simulink model "TCC_MODEL"  (R2025a)
settings: Solver=ode23t  StartTime=0.0  StopTime=1010  FixedStep=0.01  RelTol=1e-3
values from neighbouring files (symbols this model uses):
  HYST = 2    [parametros_componentes.m]
  I_table = [  1.6305773075253425 ... (first row only)    [parametros_componentes.m]
  Icc = -0.000008    (= -8e-06)    [parametros_componentes.m]
  IDD = 25e-6    (= 2.5e-05)    [parametros_componentes.m]
  Ildo = -0.00007    (= -7e-05)    [parametros_componentes.m]
  Iload = 0    [parametros_componentes.m]
  Inicio_da_descarga = 1000    [parametros_componentes.m]
  Inicio_do_curto = 10    [parametros_componentes.m]
  R_curto = 0.5    [parametros_componentes.m]
  R_descarga = (V_BATT_TOTAL+12)/corrente_Max_bat    (= 8.05)    [parametros_componentes.m]
  R_inicial = 0.18    [parametros_componentes.m]
  R_trip = 64.8    [parametros_componentes.m]
  SOC_inicial = 1    [parametros_componentes.m]
  t_table = [  93.22913720326267 ... (first row only)    [parametros_componentes.m]
  tempo_simu_curto = 70    [parametros_componentes.m]
  tempo_simu_descarga = 20    [parametros_componentes.m]
  tempo_simu_temp = 50000    [parametros_componentes.m]
  TSET = 55    [parametros_componentes.m]
  VDD = 3.3    [parametros_componentes.m]
libraries: fl_lib x29, nesl_utility x21, batt_lib x12, ee_lib x2, simulink x1, BatteryEstimators x1
(part 2 of 2)

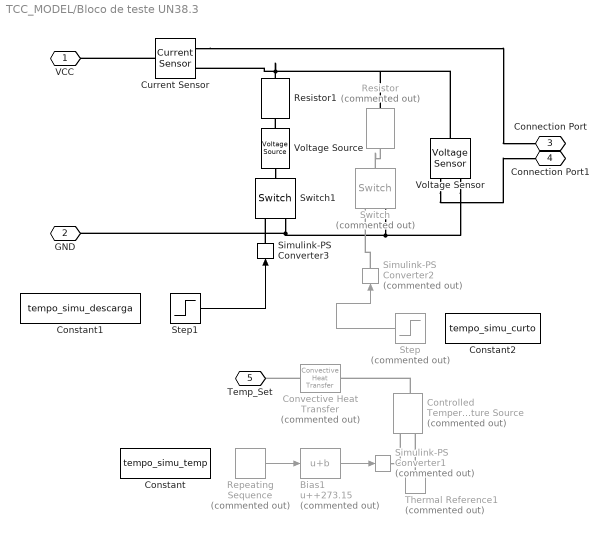
== system TCC_MODEL/Bloco de teste UN38.3 ==
  Bias1 : Bias  Commented=on  Bias=+273.15  SaturateOnIntegerOverflow=off
  Constant : Constant  Value=tempo_simu_temp
  Constant1 : Constant  Value=tempo_simu_descarga
  Constant2 : Constant  Value=tempo_simu_curto
  Controlled Temperature Source : fl_lib/Thermal/Thermal Sources/Controlled Temperature Source  Commented=on
  Convective Heat Transfer : fl_lib/Thermal/Thermal Elements/Convective Heat Transfer  Commented=on  thermal_type=foundation.enum.constant_variable.constant  area=0.03 m^2  heat_tr_coeff=10 W/(K*m^2)  min_heat_tr_coeff=1e-3 W/(K*m^2)  T_specify=off  T_priority=None  T=0 K  T_nominal_specify=off  T_nominal_value=1  T_nominal_unit=K  Q_specify=off  Q_priority=None  Q=0 W  Q_nominal_specify=off  Q_nominal_value=1  Q_nominal_unit=W
  Current Sensor : fl_lib/Electrical/Electrical Sensors/Current Sensor
  Repeating Sequence : simulink/Sources/Repeating Sequence  Commented=on  rep_seq_t=Tempo_de_teste  rep_seq_y=Valores_Temperatura
  Resistor : fl_lib/Electrical/Electrical Elements/Resistor  Commented=on  R=R_curto Ohm  i_specify=off  i_priority=None  i=0 A  i_nominal_specify=off  i_nominal_value=1  i_nominal_unit=A  v_specify=off  v_priority=None  v=0 V  v_nominal_specify=off  v_nominal_value=1  v_nominal_unit=V
  Resistor1 : fl_lib/Electrical/Electrical Elements/Resistor  R=R_descarga Ohm  i_specify=off  i_priority=None  i=0 A  i_nominal_specify=off  i_nominal_value=1  i_nominal_unit=A  v_specify=off  v_priority=None  v=0 V  v_nominal_specify=off  v_nominal_value=1  v_nominal_unit=V
  Simulink-PS Converter1 : nesl_utility/Simulink-PS Converter  Commented=on  PhysicalDomain=network_engine_domain  SubClassName=ps_input  LeftPortType=input  RightPortType=output  PseudoPeriodic=off  Frequencies=[]  NoiseDistribution=none  NoiseParameters=[]  Unit=1  AffineConversion=off  FilteringAndDerivatives=provide  SimscapeFilterOrder=1  InputFilterTimeConstant=0.001  UdotUserProvided=0
  Simulink-PS Converter2 : nesl_utility/Simulink-PS Converter  Commented=on  PhysicalDomain=network_engine_domain  SubClassName=ps_input  LeftPortType=input  RightPortType=output  PseudoPeriodic=off  Frequencies=[]  NoiseDistribution=none  NoiseParameters=[]  Unit=1  AffineConversion=off  FilteringAndDerivatives=provide  SimscapeFilterOrder=1  InputFilterTimeConstant=0.001  UdotUserProvided=0
  Simulink-PS Converter3 : nesl_utility/Simulink-PS Converter  PhysicalDomain=network_engine_domain  SubClassName=ps_input  LeftPortType=input  RightPortType=output  PseudoPeriodic=off  Frequencies=[]  NoiseDistribution=none  NoiseParameters=[]  Unit=1  AffineConversion=off  FilteringAndDerivatives=provide  SimscapeFilterOrder=1  InputFilterTimeConstant=0.001  UdotUserProvided=0
  Step : Step  Commented=on  Time=Inicio_do_curto  SampleTime=0
  Step1 : Step  Time=Inicio_da_descarga  SampleTime=0
  Switch : fl_lib/Electrical/Electrical Elements/Switch  Commented=on  R_closed=0.01 Ohm  G_open=1e-8 1/Ohm  Threshold=0.5  i_specify=off  i_priority=None  i=0 A  i_nominal_specify=off  i_nominal_value=1  i_nominal_unit=A  v_specify=off  v_priority=None  v=0 V  v_nominal_specify=off  v_nominal_value=1  v_nominal_unit=V
  Switch1 : fl_lib/Electrical/Electrical Elements/Switch  R_closed=0.01 Ohm  G_open=1e-8 1/Ohm  Threshold=0.5  i_specify=off  i_priority=None  i=0 A  i_nominal_specify=off  i_nominal_value=1  i_nominal_unit=A  v_specify=off  v_priority=None  v=0 V  v_nominal_specify=off  v_nominal_value=1  v_nominal_unit=V
  Thermal Reference1 : fl_lib/Thermal/Thermal Elements/Thermal Reference  Commented=on
  Voltage Sensor : fl_lib/Electrical/Electrical Sensors/Voltage Sensor
  Voltage Source : ee_lib/Sources/Voltage Source  dc_voltage=12 V  ac_voltage=0 V  ac_shift=0 rad  ac_frequency=60 Hz  noise_mode=ee.enum.sources.noise.Disabled  PSD=0 V^2/Hz  sample_time=1e-3 s  repeatability=ee.enum.sources.repeatability.NotRepeatable  user_seed=0  auto_seed=3922919431  i_specify=off  i_priority=None  i=0 A  i_nominal_specify=off  i_nominal_value=1  i_nominal_unit=A  v_specify=off  v_priority=None  v=0 V  v_nominal_specify=off  v_nominal_value=1  v_nominal_unit=V
  VCC : PMIOPort  Side=Left
  GND : PMIOPort  Port=2  Side=Left
  Connection Port : PMIOPort  Port=3  Side=Right
  Connection Port1 : PMIOPort  Port=4  Side=Right
  Temp_Set : PMIOPort  Port=5  Side=Right
  wires:
  Step/1 -> Simulink-PS Converter2/1
  Step1/1 -> Simulink-PS Converter3/1
  Repeating Sequence/1 -> Bias1/1
  Bias1/1 -> Simulink-PS Converter1/1
  connections:
  Voltage Sensor/RConn2 -- Switch/RConn2 -- Switch1/RConn2 -- GND/RConn1
  Simulink-PS Converter3/RConn1 -- Switch1/RConn1
  Resistor/RConn1 -- Voltage Sensor/LConn1 -- Resistor1/RConn1 -- Current Sensor/RConn2
  Switch/LConn1 -- Resistor/LConn1
  Current Sensor/RConn1 -- Connection Port/RConn1
  Simulink-PS Converter2/RConn1 -- Switch/RConn1
  Voltage Sensor/RConn1 -- Connection Port1/RConn1
  Current Sensor/LConn1 -- VCC/RConn1
  Convective Heat Transfer/RConn1 -- Temp_Set/RConn1
  Controlled Temperature Source/LConn1 -- Convective Heat Transfer/LConn1
  Simulink-PS Converter1/RConn1 -- Controlled Temperature Source/RConn1
  Thermal Reference1/LConn1 -- Controlled Temperature Source/RConn2
  Voltage Source/LConn1 -- Resistor1/LConn1
  Voltage Source/RConn1 -- Switch1/LConn1

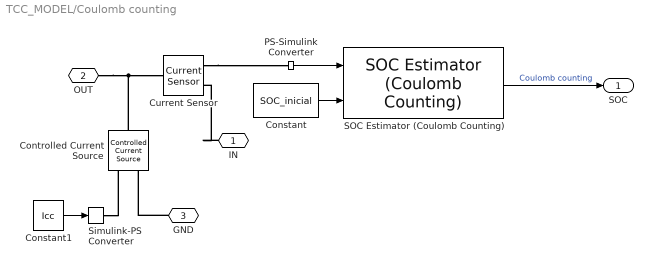
== system TCC_MODEL/Coulomb counting  ==
  Constant : Constant  Value=SOC_inicial
  Constant1 : Constant  Value=Icc
  Controlled Current Source : fl_lib/Electrical/Electrical Sources/Controlled Current Source
  Current Sensor : fl_lib/Electrical/Electrical Sensors/Current Sensor
  PS-Simulink Converter : nesl_utility/PS-Simulink Converter  PhysicalDomain=network_engine_domain  SubClassName=ps_output  LeftPortType=input  RightPortType=output  PseudoPeriodic=off  Frequencies=[]  VectorFormat=inherit  Unit=inherit  AffineConversion=off
  SOC Estimator (Coulomb Counting) : BatteryEstimators/SOC Estimator (Coulomb Counting)  CurrentInputPartition=on  AH=20  Ts=1  DataType=Inherit: auto
      settings: LibrarySourceBlock=|
      | batt_sl_lib/Estimators/SOC Estimator
      | (Coulomb Counting)
  Simulink-PS Converter : nesl_utility/Simulink-PS Converter  PhysicalDomain=network_engine_domain  SubClassName=ps_input  LeftPortType=input  RightPortType=output  PseudoPeriodic=off  Frequencies=[]  NoiseDistribution=none  NoiseParameters=[]  Unit=1  AffineConversion=off  FilteringAndDerivatives=provide  SimscapeFilterOrder=1  InputFilterTimeConstant=0.001  UdotUserProvided=0
  IN : PMIOPort  Side=Left
  OUT : PMIOPort  Port=2  Side=Right
  GND : PMIOPort  Port=3  Side=Right
  SOC : Outport
  wires:
  PS-Simulink Converter/1 -> SOC Estimator (Coulomb Counting)/1
  SOC Estimator (Coulomb Counting)/1 -> SOC/1  "Coulomb counting"
  Constant/1 -> SOC Estimator (Coulomb Counting)/2
  Constant1/1 -> Simulink-PS Converter/1
  connections:
  Current Sensor/RConn1 -- PS-Simulink Converter/LConn1
  IN/RConn1 -- Current Sensor/RConn2
  OUT/RConn1 -- Controlled Current Source/LConn1 -- Current Sensor/LConn1
  GND/RConn1 -- Controlled Current Source/RConn2
  Simulink-PS Converter/RConn1 -- Controlled Current Source/RConn1

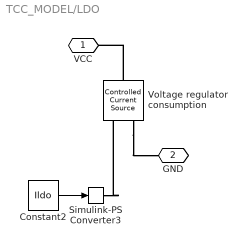
== system TCC_MODEL/LDO ==
  Constant2 : Constant  Value=Ildo
  Simulink-PS Converter3 : nesl_utility/Simulink-PS Converter  PhysicalDomain=network_engine_domain  SubClassName=ps_input  LeftPortType=input  RightPortType=output  PseudoPeriodic=off  Frequencies=[]  NoiseDistribution=none  NoiseParameters=[]  Unit=1  AffineConversion=off  FilteringAndDerivatives=provide  SimscapeFilterOrder=1  InputFilterTimeConstant=0.001  UdotUserProvided=0
  Voltage regulator consumption : fl_lib/Electrical/Electrical Sources/Controlled Current Source
  VCC : PMIOPort  Side=Left
  GND : PMIOPort  Port=2  Side=Right
  wires:
  Constant2/1 -> Simulink-PS Converter3/1
  connections:
  Simulink-PS Converter3/RConn1 -- Voltage regulator consumption/RConn1
  Voltage regulator consumption/LConn1 -- VCC/RConn1
  Voltage regulator consumption/RConn2 -- GND/RConn1

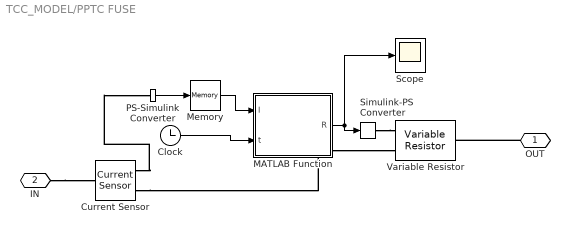
== system TCC_MODEL/PPTC FUSE ==
  Clock : Clock
  Current Sensor : fl_lib/Electrical/Electrical Sensors/Current Sensor
  MATLAB Function : MATLAB Function  TreatAsAtomicUnit=on
  Memory : Memory
  PS-Simulink Converter : nesl_utility/PS-Simulink Converter  PhysicalDomain=network_engine_domain  SubClassName=ps_output  LeftPortType=input  RightPortType=output  PseudoPeriodic=off  Frequencies=[]  VectorFormat=inherit  Unit=inherit  AffineConversion=off
  Scope : Scope
      settings: ActiveDisplayYMinimum=-7.8974999999999982  ActiveDisplayYMaximum=72.8775
  Simulink-PS Converter : nesl_utility/Simulink-PS Converter  PhysicalDomain=network_engine_domain  SubClassName=ps_input  LeftPortType=input  RightPortType=output  PseudoPeriodic=off  Frequencies=[]  NoiseDistribution=none  NoiseParameters=[]  Unit=1  AffineConversion=off  FilteringAndDerivatives=zero  SimscapeFilterOrder=1  InputFilterTimeConstant=0.001  UdotUserProvided=0
  Variable Resistor : fl_lib/Electrical/Electrical Elements/Variable Resistor  Rmin=0 Ohm  thermalEnable=false  thermal_mass=1 J/K  i_specify=off  i_priority=None  i=0 A  i_nominal_specify=off  i_nominal_value=1  i_nominal_unit=A  v_specify=off  v_priority=None  v=0 V  v_nominal_specify=off  v_nominal_value=1  v_nominal_unit=V  T_specify=off  T_priority=None  T=300 K  T_nominal_specify=off  T_nominal_value=1  T_nominal_unit=K
  OUT : PMIOPort  Side=Right
  IN : PMIOPort  Port=2  Side=Left
  wires:
  PS-Simulink Converter/1 -> Memory/1
  Memory/1 -> MATLAB Function/1(I)
  MATLAB Function/1(R) -> Scope/1, Simulink-PS Converter/1
  Clock/1 -> MATLAB Function/2(t)
  connections:
  Current Sensor/RConn2 -- Variable Resistor/LConn2
  OUT/RConn1 -- Variable Resistor/RConn1
  Simulink-PS Converter/RConn1 -- Variable Resistor/LConn1
  Current Sensor/RConn1 -- PS-Simulink Converter/LConn1
  IN/RConn1 -- Current Sensor/LConn1

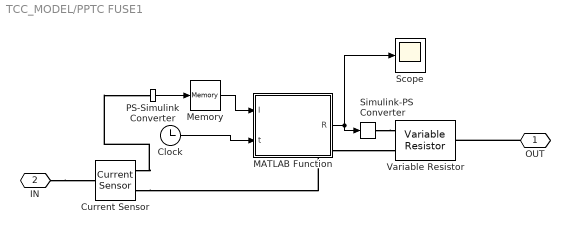
== system TCC_MODEL/PPTC FUSE1 ==
  Clock : Clock
  Current Sensor : fl_lib/Electrical/Electrical Sensors/Current Sensor
  MATLAB Function : MATLAB Function  TreatAsAtomicUnit=on
  Memory : Memory
  PS-Simulink Converter : nesl_utility/PS-Simulink Converter  PhysicalDomain=network_engine_domain  SubClassName=ps_output  LeftPortType=input  RightPortType=output  PseudoPeriodic=off  Frequencies=[]  VectorFormat=inherit  Unit=inherit  AffineConversion=off
  Scope : Scope
      settings: ActiveDisplayYMinimum=-7.8974999999999982  ActiveDisplayYMaximum=72.8775
  Simulink-PS Converter : nesl_utility/Simulink-PS Converter  PhysicalDomain=network_engine_domain  SubClassName=ps_input  LeftPortType=input  RightPortType=output  PseudoPeriodic=off  Frequencies=[]  NoiseDistribution=none  NoiseParameters=[]  Unit=1  AffineConversion=off  FilteringAndDerivatives=zero  SimscapeFilterOrder=1  InputFilterTimeConstant=0.001  UdotUserProvided=0
  Variable Resistor : fl_lib/Electrical/Electrical Elements/Variable Resistor  Rmin=0 Ohm  thermalEnable=false  thermal_mass=1 J/K  i_specify=off  i_priority=None  i=0 A  i_nominal_specify=off  i_nominal_value=1  i_nominal_unit=A  v_specify=off  v_priority=None  v=0 V  v_nominal_specify=off  v_nominal_value=1  v_nominal_unit=V  T_specify=off  T_priority=None  T=300 K  T_nominal_specify=off  T_nominal_value=1  T_nominal_unit=K
  OUT : PMIOPort  Side=Right
  IN : PMIOPort  Port=2  Side=Left
  wires:
  PS-Simulink Converter/1 -> Memory/1
  Memory/1 -> MATLAB Function/1(I)
  MATLAB Function/1(R) -> Scope/1, Simulink-PS Converter/1
  Clock/1 -> MATLAB Function/2(t)
  connections:
  Current Sensor/RConn2 -- Variable Resistor/LConn2
  OUT/RConn1 -- Variable Resistor/RConn1
  Simulink-PS Converter/RConn1 -- Variable Resistor/LConn1
  Current Sensor/RConn1 -- PS-Simulink Converter/LConn1
  IN/RConn1 -- Current Sensor/LConn1

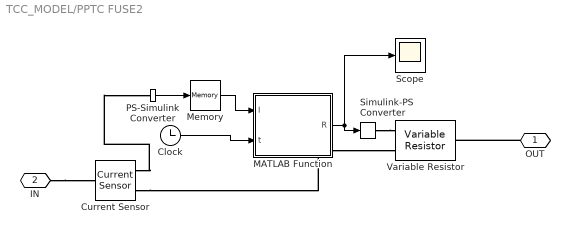
== system TCC_MODEL/PPTC FUSE2 ==
  Clock : Clock
  Current Sensor : fl_lib/Electrical/Electrical Sensors/Current Sensor
  MATLAB Function : MATLAB Function  TreatAsAtomicUnit=on
  Memory : Memory
  PS-Simulink Converter : nesl_utility/PS-Simulink Converter  PhysicalDomain=network_engine_domain  SubClassName=ps_output  LeftPortType=input  RightPortType=output  PseudoPeriodic=off  Frequencies=[]  VectorFormat=inherit  Unit=inherit  AffineConversion=off
  Scope : Scope
      settings: ActiveDisplayYMinimum=-7.8974999999999982  ActiveDisplayYMaximum=72.8775
  Simulink-PS Converter : nesl_utility/Simulink-PS Converter  PhysicalDomain=network_engine_domain  SubClassName=ps_input  LeftPortType=input  RightPortType=output  PseudoPeriodic=off  Frequencies=[]  NoiseDistribution=none  NoiseParameters=[]  Unit=1  AffineConversion=off  FilteringAndDerivatives=zero  SimscapeFilterOrder=1  InputFilterTimeConstant=0.001  UdotUserProvided=0
  Variable Resistor : fl_lib/Electrical/Electrical Elements/Variable Resistor  Rmin=0 Ohm  thermalEnable=false  thermal_mass=1 J/K  i_specify=off  i_priority=None  i=0 A  i_nominal_specify=off  i_nominal_value=1  i_nominal_unit=A  v_specify=off  v_priority=None  v=0 V  v_nominal_specify=off  v_nominal_value=1  v_nominal_unit=V  T_specify=off  T_priority=None  T=300 K  T_nominal_specify=off  T_nominal_value=1  T_nominal_unit=K
  OUT : PMIOPort  Side=Right
  IN : PMIOPort  Port=2  Side=Left
  wires:
  PS-Simulink Converter/1 -> Memory/1
  Memory/1 -> MATLAB Function/1(I)
  MATLAB Function/1(R) -> Scope/1, Simulink-PS Converter/1
  Clock/1 -> MATLAB Function/2(t)
  connections:
  Current Sensor/RConn2 -- Variable Resistor/LConn2
  OUT/RConn1 -- Variable Resistor/RConn1
  Simulink-PS Converter/RConn1 -- Variable Resistor/LConn1
  Current Sensor/RConn1 -- PS-Simulink Converter/LConn1
  IN/RConn1 -- Current Sensor/LConn1

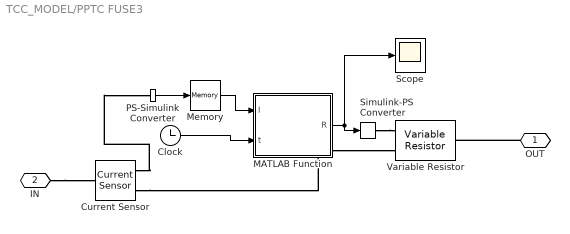
== system TCC_MODEL/PPTC FUSE3 ==
  Clock : Clock
  Current Sensor : fl_lib/Electrical/Electrical Sensors/Current Sensor
  MATLAB Function : MATLAB Function  TreatAsAtomicUnit=on
  Memory : Memory
  PS-Simulink Converter : nesl_utility/PS-Simulink Converter  PhysicalDomain=network_engine_domain  SubClassName=ps_output  LeftPortType=input  RightPortType=output  PseudoPeriodic=off  Frequencies=[]  VectorFormat=inherit  Unit=inherit  AffineConversion=off
  Scope : Scope
      settings: ActiveDisplayYMinimum=-7.8974999999999982  ActiveDisplayYMaximum=72.8775
  Simulink-PS Converter : nesl_utility/Simulink-PS Converter  PhysicalDomain=network_engine_domain  SubClassName=ps_input  LeftPortType=input  RightPortType=output  PseudoPeriodic=off  Frequencies=[]  NoiseDistribution=none  NoiseParameters=[]  Unit=1  AffineConversion=off  FilteringAndDerivatives=zero  SimscapeFilterOrder=1  InputFilterTimeConstant=0.001  UdotUserProvided=0
  Variable Resistor : fl_lib/Electrical/Electrical Elements/Variable Resistor  Rmin=0 Ohm  thermalEnable=false  thermal_mass=1 J/K  i_specify=off  i_priority=None  i=0 A  i_nominal_specify=off  i_nominal_value=1  i_nominal_unit=A  v_specify=off  v_priority=None  v=0 V  v_nominal_specify=off  v_nominal_value=1  v_nominal_unit=V  T_specify=off  T_priority=None  T=300 K  T_nominal_specify=off  T_nominal_value=1  T_nominal_unit=K
  OUT : PMIOPort  Side=Right
  IN : PMIOPort  Port=2  Side=Left
  wires:
  PS-Simulink Converter/1 -> Memory/1
  Memory/1 -> MATLAB Function/1(I)
  MATLAB Function/1(R) -> Scope/1, Simulink-PS Converter/1
  Clock/1 -> MATLAB Function/2(t)
  connections:
  Current Sensor/RConn2 -- Variable Resistor/LConn2
  OUT/RConn1 -- Variable Resistor/RConn1
  Simulink-PS Converter/RConn1 -- Variable Resistor/LConn1
  Current Sensor/RConn1 -- PS-Simulink Converter/LConn1
  IN/RConn1 -- Current Sensor/LConn1

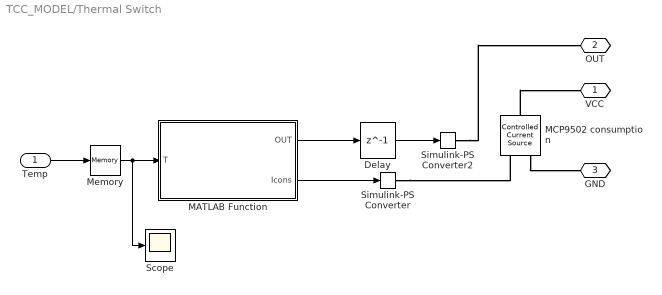
== system TCC_MODEL/Thermal Switch ==
  Temp : Inport
  Delay : Delay  DelayLength=1  InputProcessing=Columns as channels (frame based)
  MATLAB Function : MATLAB Function  TreatAsAtomicUnit=on
  MCP9502 consumption : fl_lib/Electrical/Electrical Sources/Controlled Current Source
  Memory : Memory
  Scope : Scope
      settings: ActiveDisplayYMinimum=-132.4386075017589  ActiveDisplayYMaximum=261.474881625119  DataLoggingVariableName=ScopeData5
  Simulink-PS Converter : nesl_utility/Simulink-PS Converter  PhysicalDomain=network_engine_domain  SubClassName=ps_input  LeftPortType=input  RightPortType=output  PseudoPeriodic=off  Frequencies=[]  NoiseDistribution=none  NoiseParameters=[]  Unit=1  AffineConversion=off  FilteringAndDerivatives=provide  SimscapeFilterOrder=1  InputFilterTimeConstant=0.001  UdotUserProvided=0
  Simulink-PS Converter2 : nesl_utility/Simulink-PS Converter  PhysicalDomain=network_engine_domain  SubClassName=ps_input  LeftPortType=input  RightPortType=output  PseudoPeriodic=off  Frequencies=[]  NoiseDistribution=none  NoiseParameters=[]  Unit=1  AffineConversion=off  FilteringAndDerivatives=provide  SimscapeFilterOrder=1  InputFilterTimeConstant=0.001  UdotUserProvided=0
  VCC : PMIOPort  Side=Left
  OUT : PMIOPort  Port=2  Side=Left
  GND : PMIOPort  Port=3  Side=Right
  wires:
  MATLAB Function/2(Icons) -> Simulink-PS Converter/1
  Temp/1 -> Memory/1
  Memory/1 -> Scope/1, MATLAB Function/1(T)
  Delay/1 -> Simulink-PS Converter2/1
  MATLAB Function/1(OUT) -> Delay/1
  connections:
  MCP9502 consumption/LConn1 -- VCC/RConn1
  Simulink-PS Converter/RConn1 -- MCP9502 consumption/RConn1
  MCP9502 consumption/RConn2 -- GND/RConn1
  Simulink-PS Converter2/RConn1 -- OUT/RConn1

== matlab function TCC_MODEL/Thermal Switch/MATLAB Function ==
  data: OUT output; T input; Icons output; VDD parameter; TSET parameter; HYST parameter; IDD parameter; Iload parameter
function [OUT, Icons] = MCP9502_func(T,VDD,TSET, HYST, IDD, Iload)

T = T(1);

persistent estado

if isempty(estado)
    estado = 0;
end

if estado == 0 && T >= TSET
    estado = 1;
elseif estado == 1 && T <= (TSET - HYST)
    estado = 0;
end

OUT = (1 - estado) * VDD;

if estado == 1
    Icons = -(IDD + Iload);
else
    Icons = -IDD;
end

end

== matlab function TCC_MODEL/PPTC FUSE/MATLAB Function ==
  settings: updateMethod=DISCRETE
  data: I input; R output; t input; R_inicial parameter; I_table parameter; t_table parameter; R_trip parameter
function R = PPTC_tabela(I,t,R_inicial,I_table, t_table, R_trip)

I = I(1);
t = t(1);

persistent tempo_acima disparado t_anterior

if isempty(tempo_acima)
    tempo_acima = 0;
    disparado = false;
    t_anterior = t;
end

dt = t - t_anterior;

if dt < 0
    dt = 0;
end

t_anterior = t;

I_abs = abs(I);

if ~disparado

    if I_abs < I_table(1)

        tempo_acima = 0;

    else

        if I_abs >= I_table(end)
            t_trip_atual = t_table(end);
        else
            t_trip_atual = exp(interp1(log(I_table), log(t_table), log(I_abs)));
        end

        tempo_acima = tempo_acima + dt;

        if tempo_acima >= t_trip_atual
            disparado = true;
        end
    end
end

if disparado
    R = R_trip;
else
    R = R_inicial;
end

if R < 0.01
    R = 0.01;
end

if R > 1e6
    R = 1e6;
end

end

== matlab function TCC_MODEL/PPTC FUSE1/MATLAB Function ==
  settings: updateMethod=DISCRETE
  data: I input; R output; t input; R_inicial parameter; I_table parameter; t_table parameter; R_trip parameter
function R = PPTC_tabela(I,t,R_inicial,I_table, t_table, R_trip)

I = I(1);
t = t(1);

persistent tempo_acima disparado t_anterior

if isempty(tempo_acima)
    tempo_acima = 0;
    disparado = false;
    t_anterior = t;
end

dt = t - t_anterior;

if dt < 0
    dt = 0;
end

t_anterior = t;

I_abs = abs(I);

if ~disparado

    if I_abs < I_table(1)

        tempo_acima = 0;

    else

        if I_abs >= I_table(end)
            t_trip_atual = t_table(end);
        else
            t_trip_atual = exp(interp1(log(I_table), log(t_table), log(I_abs)));
        end

        tempo_acima = tempo_acima + dt;

        if tempo_acima >= t_trip_atual
            disparado = true;
        end
    end
end

if disparado
    R = R_trip;
else
    R = R_inicial;
end

if R < 0.01
    R = 0.01;
end

if R > 1e6
    R = 1e6;
end

end

== matlab function TCC_MODEL/PPTC FUSE2/MATLAB Function ==
  settings: updateMethod=DISCRETE
  data: I input; R output; t input; R_inicial parameter; I_table parameter; t_table parameter; R_trip parameter
function R = PPTC_tabela(I,t,R_inicial,I_table, t_table, R_trip)

I = I(1);
t = t(1);

persistent tempo_acima disparado t_anterior

if isempty(tempo_acima)
    tempo_acima = 0;
    disparado = false;
    t_anterior = t;
end

dt = t - t_anterior;

if dt < 0
    dt = 0;
end

t_anterior = t;

I_abs = abs(I);

if ~disparado

    if I_abs < I_table(1)

        tempo_acima = 0;

    else

        if I_abs >= I_table(end)
            t_trip_atual = t_table(end);
        else
            t_trip_atual = exp(interp1(log(I_table), log(t_table), log(I_abs)));
        end

        tempo_acima = tempo_acima + dt;

        if tempo_acima >= t_trip_atual
            disparado = true;
        end
    end
end

if disparado
    R = R_trip;
else
    R = R_inicial;
end

if R < 0.01
    R = 0.01;
end

if R > 1e6
    R = 1e6;
end

end

== matlab function TCC_MODEL/PPTC FUSE3/MATLAB Function ==
  settings: updateMethod=DISCRETE
  data: I input; R output; t input; R_inicial parameter; I_table parameter; t_table parameter; R_trip parameter
function R = PPTC_tabela(I,t,R_inicial,I_table, t_table, R_trip)

I = I(1);
t = t(1);

persistent tempo_acima disparado t_anterior

if isempty(tempo_acima)
    tempo_acima = 0;
    disparado = false;
    t_anterior = t;
end

dt = t - t_anterior;

if dt < 0
    dt = 0;
end

t_anterior = t;

I_abs = abs(I);

if ~disparado

    if I_abs < I_table(1)

        tempo_acima = 0;

    else

        if I_abs >= I_table(end)
            t_trip_atual = t_table(end);
        else
            t_trip_atual = exp(interp1(log(I_table), log(t_table), log(I_abs)));
        end

        tempo_acima = tempo_acima + dt;

        if tempo_acima >= t_trip_atual
            disparado = true;
        end
    end
end

if disparado
    R = R_trip;
else
    R = R_inicial;
end

if R < 0.01
    R = 0.01;
end

if R > 1e6
    R = 1e6;
end

end
